simulink model "f123"  (R2016b)
settings: Solver=ode4  StartTime=0.0  StopTime=inf  FixedStep=0.002  RelTol=1e-3  EnableMultiTasking=on
undefined symbols (not defined in the file or in its folder): bit, Standard
libraries: slrtlib x3, slrtsoftinglib x3, dsparch4 x1
settings Model: xpc_rtwmakecfg_data=_xpccanac2pci_  SimulationMode=external  Creator=Administrator  LastModifiedBy=Administrator
settings SolverCC: EnableConcurrentExecution=on
settings DataIOCC: SaveFormat=StructureWithTime
settings OptimizationCC: BlockReduction=off  OptimizeBlockIOStorage=off  BufferReuse=off  GlobalBufferReuse=off  ExpressionFolding=off  LocalBlockOutputs=off
settings HardwareCC: ProdBitPerPointer=32  ProdBitPerSizeT=32  ProdBitPerPtrDiffT=32  ProdLargestAtomicFloat=None  ProdWordSize=32  ProdLongLongMode=on  ProdHWDeviceType=Generic->32-bit x86 compatible
settings RTWCC: SystemTargetFile=slrt.tlc  TemplateMakefile=slrt_default_tmf  Description=Simulink Real-Time  RTWCompilerOptimization=on

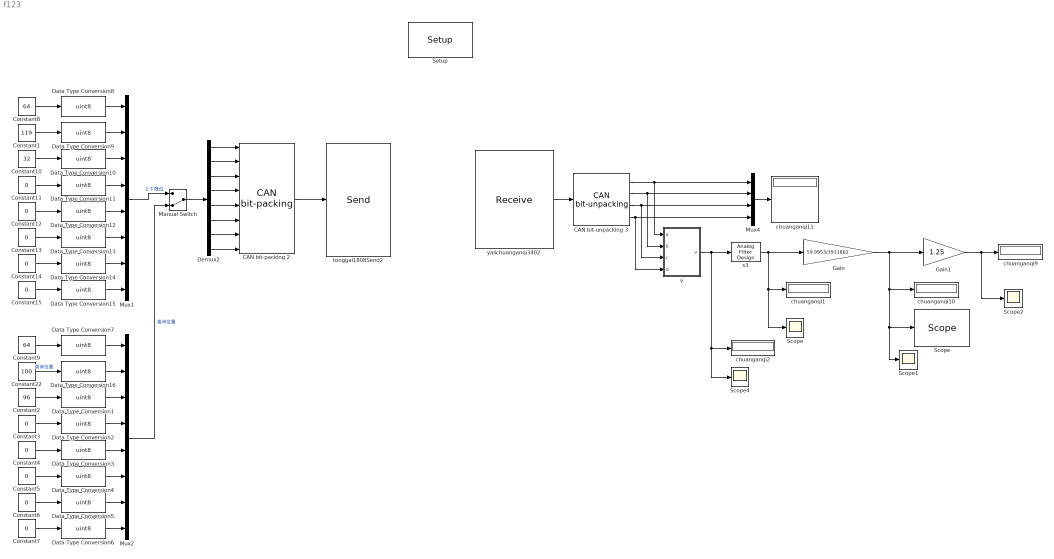
== system f123 ==
  CAN bit-packing 2 : slrtlib/CAN/Utilities/CAN bit-packing   bitpatterns={ [0:7] [8:15] [16:23] [24:31] [32:39] [40:47] [48:55] [56:63]}
  CAN bit-unpacking 3 : slrtlib/CAN/Utilities/CAN bit-unpacking   bitpatterns={ [32:39],[40:47],[48:55],[56:63] }  dtypes={ 'uint8','uint8','uint8','uint8' }
  Constant1 : Constant  Value=119
  Constant10 : Constant  Value=32
  Constant{3..7,11..15} (10 alike) : Constant  Value=0
  Constant2 : Constant  Value=96
  Constant22 : Constant  Value=100
  Constant8 : Constant  Value=64
  Constant9 : Constant  Value=64
  Data Type Conversion{1..16} (16 alike) : DataTypeConversion  OutDataTypeStr=uint8
  Demux2 : Demux  Outputs=8
  Gain : Gain  Gain=59.9953/3931862
  Gain1 : Gain  Gain=1.25
  Manual Switch : ManualSwitch  CurrentSetting=0
  Mux1 : Mux  Inputs=8
  Mux2 : Mux  Inputs=8
  Mux4 : Mux
  Scope{,1..2,4} (4 alike) : Scope
  "Scope " : slrtlib/Displays and Logging/Scope   scopeno=1  scopetype=Target  autostart=on  viewmode=Graphical redraw  formatstr='%15.6f'  grid=on  ylimits=[0,0]  nosamples=250  noprepostsamples=0  interleave=1  triggermode=FreeRun  triggersignal=1  trigsignalfromport=off  triggerlevel=0.0  triggerslope=Either  triggerscope=1  triggersample=0  filename=data.dat  mode=Lazy  writesize=512  autorestart=off  dynamicfilemode=off  maxwritefilesize=512*1024^2
  "Setup " : slrtsoftinglib/CAN-AC2-PCI SJA 1000/Setup   board=1  can1bus=Highspeed (ISO 11898)  can1Baudrate=1 MBaud  can1UserBR=[1,1,4,3]  can2bus=Highspeed (ISO 11898)  can2Baudrate=1 MBaud  can2UserBR=[1,1,4,3]  init=[]  term=[]  bus_off_out=off  bus_off_rec=Off  ioBaseAddress=-1
  chuanganqi{1..2,9..11} (5 alike) : Display
  s3 : dsparch4/Analog Filter Design  method=Butterworth  filttype=Lowpass  N=1  Wlo=10  Whi=80  Rp=2  Rs=40
  tonggai1808Send2 : slrtsoftinglib/CAN-AC2-PCI SJA 1000/Send   board=1  canPort=CAN 2  range=Standard (11-bit)  ids=1537  sizes=[8]  output=off  ts=-1  ididx=[0]
  v : MATLAB Function  TreatAsAtomicUnit=on
  yalichuanganqi3402 : slrtsoftinglib/CAN-AC2-PCI SJA 1000/Receive   board=1  canPort=CAN 2  range=Standard (11-bit)  ids=1409  lengths=8  output=Data  inten=off  ts=-1  ididx=[0]
  wires:
  Demux2/3 -> CAN bit-packing 2/3
  Demux2/7 -> CAN bit-packing 2/7
  Demux2/8 -> CAN bit-packing 2/8
  Demux2/1 -> CAN bit-packing 2/1
  Demux2/2 -> CAN bit-packing 2/2
  Demux2/4 -> CAN bit-packing 2/4
  Demux2/5 -> CAN bit-packing 2/5
  Demux2/6 -> CAN bit-packing 2/6
  CAN bit-packing 2/1 -> tonggai1808Send2/1
  Data Type Conversion14/1 -> Mux1/7
  Data Type Conversion8/1 -> Mux1/1
  Data Type Conversion9/1 -> Mux1/2
  Data Type Conversion10/1 -> Mux1/3
  Data Type Conversion11/1 -> Mux1/4
  Data Type Conversion12/1 -> Mux1/5
  Data Type Conversion13/1 -> Mux1/6
  Constant13/1 -> Data Type Conversion13/1
  Constant8/1 -> Data Type Conversion8/1
  Constant11/1 -> Data Type Conversion11/1
  Constant12/1 -> Data Type Conversion12/1
  Constant14/1 -> Data Type Conversion14/1
  Constant15/1 -> Data Type Conversion15/1
  Constant10/1 -> Data Type Conversion10/1
  Data Type Conversion15/1 -> Mux1/8
  Mux1/1 -> Manual Switch/1  "上下限位"
  Constant1/1 -> Data Type Conversion9/1
  Data Type Conversion5/1 -> Mux2/7
  Data Type Conversion7/1 -> Mux2/1
  Data Type Conversion16/1 -> Mux2/2
  Data Type Conversion1/1 -> Mux2/3
  Data Type Conversion2/1 -> Mux2/4
  Data Type Conversion3/1 -> Mux2/5
  Data Type Conversion4/1 -> Mux2/6
  Constant5/1 -> Data Type Conversion4/1
  Constant9/1 -> Data Type Conversion7/1
  Constant3/1 -> Data Type Conversion2/1
  Constant4/1 -> Data Type Conversion3/1
  Constant6/1 -> Data Type Conversion5/1
  Constant7/1 -> Data Type Conversion6/1
  Constant2/1 -> Data Type Conversion1/1
  Data Type Conversion6/1 -> Mux2/8
  Mux2/1 -> Manual Switch/2  "查询位置"
  Constant22/1 -> Data Type Conversion16/1  "查询位置"
  Manual Switch/1 -> Demux2/1
  yalichuanganqi3402/1 -> CAN bit-unpacking 3/1
  Mux4/1 -> chuanganqi11/1
  CAN bit-unpacking 3/1 -> v/1(a), Mux4/1
  CAN bit-unpacking 3/2 -> v/2(b), Mux4/2
  CAN bit-unpacking 3/3 -> v/3(c), Mux4/3
  CAN bit-unpacking 3/4 -> v/4(d), Mux4/4
  Gain/1 -> Scope1/1, "Scope "/1, chuanganqi10/1, Gain1/1
  v/1(v) -> Scope4/1, chuanganqi2/1, s3/1
  s3/1 -> Gain/1, Scope/1, chuanganqi1/1
  Gain1/1 -> Scope2/1, chuanganqi9/1

== matlab function f123/v ==
  data: a input; v output; b input; c input; d input
function v  = velocity(a, b, c, d)
A = dec2bin(a);
B = dec2bin(b);
C = dec2bin(c);
D = dec2bin(d);

BASE = '00000000';
LA = length(A);
for i = 1:LA
    BASE(8-LA+i) = A(i);
end
A = BASE;

BASE = '00000000';
LB = length(B);
for i = 1:LB
    BASE(8-LB+i) = B(i);
end
B = BASE;

BASE = '00000000';
LC = length(C);
for i = 1:LC
    BASE(8-LC+i) = C(i);
end
C = BASE;

BASE = '00000000';
LD = length(D);
for i = 1:LD
    BASE(8-LD+i) = D(i);
end
D = BASE;

Vbin = [D, C, B, A];
V = bin2dec(Vbin);
if d < 128  %bin2dec('10000000')=128
    v = V;
else
    V = V-1;
    v = -(4294967295 - V); %bin2dec('11111111111111111111111111111111')（一共32位）=4294967295
end
